simulink model "H_inf_incompleto"  (R2024a)
settings: Solver=VariableStepAuto  StartTime=0.0  StopTime=200  RelTol=1e-3
values from neighbouring files (symbols this model uses):
  den_G = [1 betaF/J + (Lb*m_b+Lm*m_m)*g*cosd(theta_ref)/J]    [Proyecto_Hinf_incompleto.m]
  K = K    [Proyecto_Hinf_incompleto.m]
  num_G = 21*Kf*Lm/J    (= 23.7352730289)    [Proyecto_Hinf_incompleto.m]
libraries: simulink x1
settings Model: Creator=PERSONAL  LastModifiedBy=alfar
settings RTWCC: GPUComputeCapability=3.5

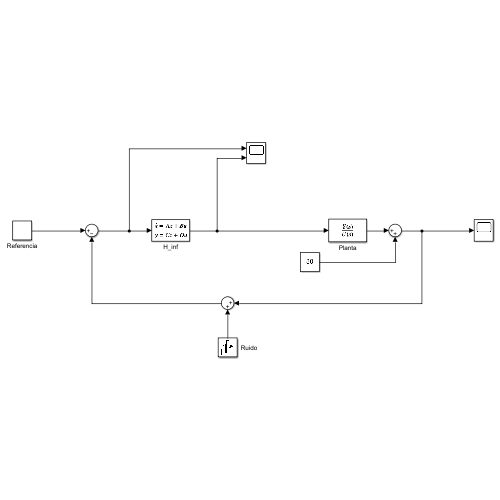
[thumbnail: Simulink's stored preview of the top-level diagram]
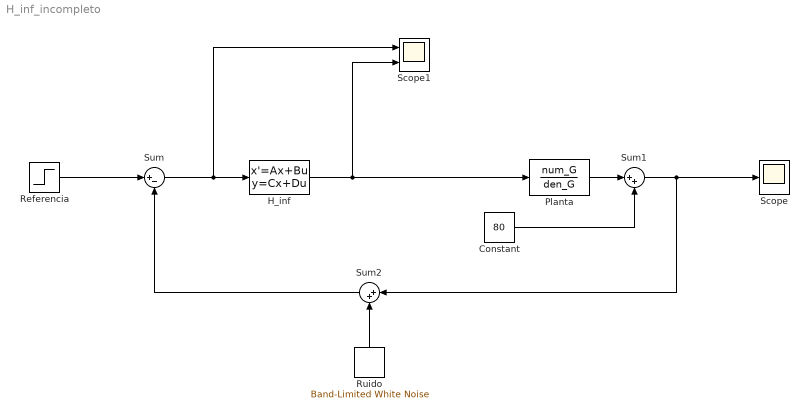
== system H_inf_incompleto ==
  Constant : Constant  Value=80
  H_inf : StateSpace  A=K.A  B=K.B  C=K.C  D=K.D  InitialCondition=0
  Planta : TransferFcn  Numerator=num_G  Denominator=den_G
  Referencia : Step  After=20  SampleTime=0
  Ruido : simulink/Sources/Band-Limited White Noise  Cov=[0]  Ts=0.1  seed=[23341]
  Scope : Scope
  Scope1 : Scope  NumInputPorts=2
  Sum : Sum  Inputs=|+-
  Sum1 : Sum  Inputs=|++
  Sum2 : Sum  Inputs=|++
  wires:
  Referencia/1 -> Sum/1
  Sum/1 -> Scope1/1, H_inf/1
  H_inf/1 -> Planta/1, Scope1/2
  Constant/1 -> Sum1/2
  Ruido/1 -> Sum2/2
  Sum2/1 -> Sum/2
  Planta/1 -> Sum1/1
  Sum1/1 -> Sum2/1, Scope/1
